simulink model "Simulink_Grid_Scale_Challenges_&_Solutions_for_Integrating_500_GW_Renewable_Energy_into_the_Indian_Power_System_by_2030"  (R2024a)
settings: Solver=VariableStepAuto  StartTime=0.0  StopTime=10.0  RelTol=1e-3
undefined symbols (not defined in the file): DiscIntNeverNeededParam, droopP1, droopP2, droopQ1, droopQ2, Ts, Ts_AC
libraries: nesl_utility x29, fl_lib x28, ee_lib x22, spsFourierLib x2, simulink x1
(part 2 of 2)

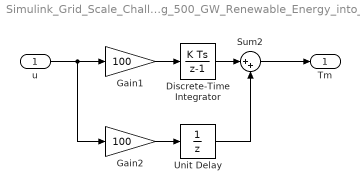
== system Simulink_Grid_Scale_Challenges_&_Solutions_for_Integrating_500_GW_Renewable_Energy_into_the_Indian_Power_System_by_2030/Generator1/Prime mover and governor/speed control ==
  u : Inport
  Discrete-Time Integrator : DiscreteIntegrator  gainval=1  InitialCondition=0.1  SampleTime=-1  ICPrevOutput=DiscIntNeverNeededParam  ICPrevScaledInput=DiscIntNeverNeededParam
  Gain1 : Gain  Gain=100
  Gain2 : Gain  Gain=100
  Sum2 : Sum  Inputs=|++
  Unit Delay : UnitDelay  SampleTime=-1  HasFrameUpgradeWarning=on
  Tm : Outport
  wires:
  Gain2/1 -> Unit Delay/1
  u/1 -> Gain1/1, Gain2/1
  Discrete-Time Integrator/1 -> Sum2/1
  Gain1/1 -> Discrete-Time Integrator/1
  Unit Delay/1 -> Sum2/2
  Sum2/1 -> Tm/1

== system Simulink_Grid_Scale_Challenges_&_Solutions_for_Integrating_500_GW_Renewable_Energy_into_the_Indian_Power_System_by_2030/Generator2/AVR and exciter/Subsystem1 ==
  In1 : Inport
  Discrete-Time Integrator : DiscreteIntegrator  gainval=20  SampleTime=-1  ICPrevOutput=DiscIntNeverNeededParam  ICPrevScaledInput=DiscIntNeverNeededParam
  Sum : Sum  Inputs=|+-
  Out1 : Outport
  wires:
  In1/1 -> Sum/1
  Discrete-Time Integrator/1 -> Out1/1, Sum/2
  Sum/1 -> Discrete-Time Integrator/1

== system Simulink_Grid_Scale_Challenges_&_Solutions_for_Integrating_500_GW_Renewable_Energy_into_the_Indian_Power_System_by_2030/Generator2/AVR and exciter/voltage conrtrol ==
  u : Inport
  Discrete-Time Integrator : DiscreteIntegrator  InitialCondition=1  SampleTime=-1  ICPrevOutput=DiscIntNeverNeededParam  ICPrevScaledInput=DiscIntNeverNeededParam
  Gain : Gain  Gain=500
  Gain1 : Gain  Gain=1000
  Sum1 : Sum  Inputs=|++
  Unit Delay : UnitDelay  SampleTime=-1  HasFrameUpgradeWarning=on
  Efd : Outport
  wires:
  Sum1/1 -> Efd/1
  Unit Delay/1 -> Sum1/2
  Gain1/1 -> Unit Delay/1
  Gain/1 -> Discrete-Time Integrator/1
  u/1 -> Gain/1, Gain1/1
  Discrete-Time Integrator/1 -> Sum1/1

== system Simulink_Grid_Scale_Challenges_&_Solutions_for_Integrating_500_GW_Renewable_Energy_into_the_Indian_Power_System_by_2030/Generator2/Prime mover and governor/Subsystem1 ==
  In1 : Inport
  Discrete-Time Integrator : DiscreteIntegrator  gainval=20  SampleTime=-1  ICPrevOutput=DiscIntNeverNeededParam  ICPrevScaledInput=DiscIntNeverNeededParam
  Sum : Sum  Inputs=|+-
  Out1 : Outport
  wires:
  In1/1 -> Sum/1
  Discrete-Time Integrator/1 -> Out1/1, Sum/2
  Sum/1 -> Discrete-Time Integrator/1

== system Simulink_Grid_Scale_Challenges_&_Solutions_for_Integrating_500_GW_Renewable_Energy_into_the_Indian_Power_System_by_2030/Generator2/Prime mover and governor/speed control ==
  u : Inport
  Discrete-Time Integrator : DiscreteIntegrator  gainval=1  InitialCondition=0.1  SampleTime=-1  ICPrevOutput=DiscIntNeverNeededParam  ICPrevScaledInput=DiscIntNeverNeededParam
  Gain1 : Gain  Gain=100
  Gain2 : Gain  Gain=100
  Sum2 : Sum  Inputs=|++
  Unit Delay : UnitDelay  SampleTime=-1  HasFrameUpgradeWarning=on
  Tm : Outport
  wires:
  Sum2/1 -> Tm/1
  Unit Delay/1 -> Sum2/2
  Gain1/1 -> Discrete-Time Integrator/1
  Discrete-Time Integrator/1 -> Sum2/1
  u/1 -> Gain2/1, Gain1/1
  Gain2/1 -> Unit Delay/1

== matlab function Simulink_Grid_Scale_Challenges_&_Solutions_for_Integrating_500_GW_Renewable_Energy_into_the_Indian_Power_System_by_2030/Solar/MPPT Algorithm/MPPT Algorithm ==
  settings: updateMethod=DISCRETE  sampleTime=Ts_DC
  data: Param input; V input; I input; D output
function D  = PandO(Param, V, I)

% MPPT controller based on the Perturb & Observe algorithm.

% D output = Duty cycle of the boost converter (value between 0 and 1)
%
% V input = PV array terminal voltage (V)
% I input = PV array current (A)
%
% Param input:
Dinit = Param(1);  %Initial value for D output
Dmax = Param(2);   %Maximum value for D
Dmin = Param(3);   %Minimum value for D
deltaD = Param(4); %Increment value used to increase/decrease the duty cycle D
% ( increasing D = decreasing Vref )
%  

persistent Vold Pold Dold;

if isempty(Vold)
    Vold=0;
    Pold=0;
    Dold=Dinit;
end
P= V*I;
dV= V - Vold;
dP= P - Pold;

if dP ~= 0
    %     if dP>1e-9  & dP<-1e-9 & Enabled ~=0
    if dP < 0
        if dV < 0
            D = Dold - deltaD;
        else
            D = Dold + deltaD;
        end
    else
        if dV < 0
            D = Dold + deltaD;
        else
            D = Dold - deltaD;
        end
    end
else
    D = Dold;
end

if D >= Dmax || D<= Dmin
    D = Dold;
end

Dold = D;
Vold = V;
Pold = P;
